simulink model "sim12ex6"  (Simulink 4.00)
settings: Solver=ode45  SolverMode=SingleTasking  StartTime=0.0  StopTime=20  MaxStep=.10  RelTol=1e-3  AbsTol=1e-3
settings Model: LastModifiedBy=saadat  SaveTime=off  SaveOutput=off  LimitDataPoints=off  RTWTemplateMakefile=grt_vc.tmf  ExtModeTrigMode=oneshot  ExtModeArmWhenConnect=off

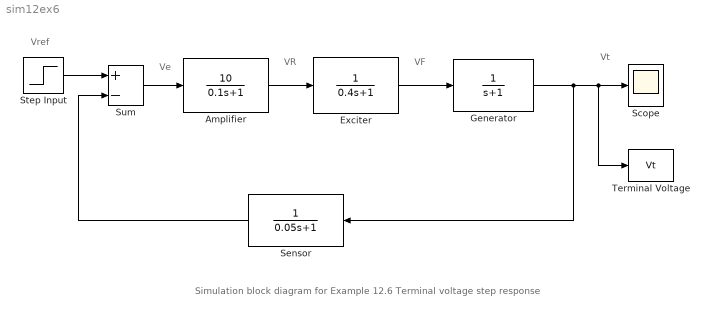
== system sim12ex6 ==
  note: Simulation block diagram for Example 12.6
      | Terminal voltage step response
  note: Vt
  note: VF
  note: VR
  note: Ve
  note: Vref
  Amplifier : TransferFcn  Numerator=[10]  Denominator="[0.1  1]"  AbsoluteTolerance=auto  Realization=auto
  Exciter : TransferFcn  Numerator=[1]  Denominator="[0.4  1]"  AbsoluteTolerance=auto  Realization=auto
  Generator : TransferFcn  Numerator=[1]  Denominator="[1  1]"  AbsoluteTolerance=auto  Realization=auto
  Scope : Scope
      settings: TickLabels=on  TimeRange=20  YMin=0  YMax=2  SaveToWorkspace=off  SaveName=ScopeData  DataFormat=Array  LimitDataPoints=on  MaxDataPoints=5000
  Sensor : TransferFcn  Orientation=left  Numerator=[1]  Denominator="[0.05  1]"  AbsoluteTolerance=auto  Realization=auto
  Step Input : Step  Time=0  Before=0  After=1  SampleTime=0
  Sum : Sum  Inputs=+-  SaturateOnIntegerOverflow=on
  Terminal Voltage : ToWorkspace  VariableName=Vt  SampleTime=0  SaveFormat=Array
      settings: MaxDataPoints=1000
  wires:
  Generator/1 -> Terminal Voltage/1, Scope/1, Sensor/1
  Sensor/1 -> Sum/2
  Exciter/1 -> Generator/1
  Amplifier/1 -> Exciter/1
  Sum/1 -> Amplifier/1
  Step Input/1 -> Sum/1
